simulink library "XXCopter_Control"  (R2015a)
settings: Solver=ode45  SolverMode=SingleTasking  StartTime=0.0  StopTime=10.0  RelTol=1e-3
undefined symbols (not defined in the file or in its folder): a, C_d0, h, h_FA, h_M, I_prop, I_tube, J_FA, J_T, m_FA, m_M, m_prop, Newton, omega_n, R, Raphson, rho, sigma, T_ctrl, theta_0, theta_1, Throtle_TTO_vec, TO_map_Omega, TO_map_Throtle, v_i0, v_i_adim, Vx_adim, Vz_adim, xi
undefined symbols (not defined in the file): direct_feedforward, l, l_arm, Rotation_sign, T_sim
libraries: vrlib x16, XXCopter_Control x10, aerolibutil x3, qcatlib x1, dspinverses x1
(part 1 of 2)
settings Model: Creator=David  LastModifiedBy=David
settings OptimizationCC: BlockReduction=off  BooleanDataType=off
settings DebuggingCC: SaveWithParameterizedLinksMsg=none  UnderspecifiedInitializationDetection=Classic  MergeDetectMultiDrivingBlocksExec=none  SignalResolutionControl=TryResolveAllWithWarning  StrictBusMsg=Warning
settings HardwareCC: TargetUnknown=on

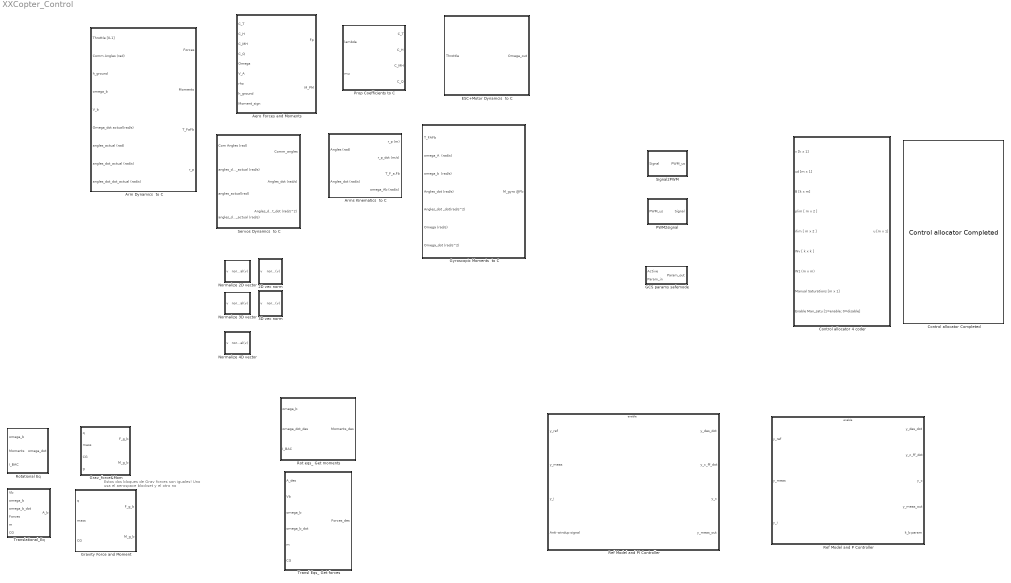
== system XXCopter_Control ==
  note: Estos dos bloques de Grav forces son iguales!
      | Uno usa el aerospace blockset y el otro no
  2D vec norm : Subsystem  TreatAsAtomicUnit=on
  3D vec norm : Subsystem  TreatAsAtomicUnit=on
  "Aero Forces and Moments " : Subsystem  TreatAsAtomicUnit=on
  Arm Dynamics  to C : Subsystem  TreatAsAtomicUnit=on  mask(Arm dynamics, kinematics, forces and moments){Rot_sign=Rotation_sign(1), arm_hub_pos=l*[1;0;0], Arm_axis=[l_arm;0;0], arm_num=1, eta_dir=[1;0;0], gamma_dir=[0;1;0], J_T=J_T, J_FA=J_FA, h=h, switch_val=direct_feedforward, omega_n=35, xi=1.45, eta_inf_lim=deg2rad(-180), eta_sup_lim=deg2rad(180), gamma_inf_lim=deg2rad(-90), gamma_sup_lim=deg2rad(30)}
      mask prompts: Rot_sign "Rotation Sign"; arm_hub_pos "Arm Hub position"; Arm_axis "Arm Hub from servo"; arm_num "Arm number"; eta_dir "eta direcction"; gamma_dir "gamma direction"; J_T "Inertia Motor+prop"; J_FA "Inertia Forearm"; h "h propeller hub"; switch_val "Generation method"; omega_n "Servo natural frequency"; xi "Servo damping"; eta_inf_lim "Pan Servo inf lim (rad)"; eta_sup_lim "Pan Servo sup lim (rad)"; gamma_inf_lim "Tilt Servo inf lim (rad)"; gamma_sup_lim "Tilt servo sup lim  (rad)"
      mask help:
      | This block only accepts arms oriented in x-axis or y-axis: eta and gamma directions can only be [1,0,0] or [0,1,0]
      | Note rotations order is [eta (pan) ,gamma (tilt),0]
      |
      | If Arm number 1 (Forward one)
      | eta_dir=[1,0,0]
      | gamma_dir=[0,1,0]
      |
      | If Arm number 2 or 3 (rear ones)
      | eta_dir=[0,1,0]
      | gamma_dir=[1,0,0]
      mask TypeOptions Rot_sign: Aerodynamics Propeller/Rot_sign | Gyroscopic Moments  to C/Rot_sign
      mask TypeOptions arm_hub_pos: Arms Kinematics  to C/Arm_hub_position
      mask TypeOptions Arm_axis: Gyroscopic Moments  to C/Arm_axis
      mask TypeOptions arm_num: Arms Kinematics  to C/Arm_number
      mask TypeOptions eta_dir: Arms Kinematics  to C/eta_dir | Gyroscopic Moments  to C/eta_dir
      mask TypeOptions gamma_dir: Arms Kinematics  to C/gamma_dir | Gyroscopic Moments  to C/gamma_dir
      mask TypeOptions J_T: Gyroscopic Moments  to C/J_T
      mask TypeOptions J_FA: Gyroscopic Moments  to C/J_FA
      mask TypeOptions h: Arms Kinematics  to C/h_prop
      mask TypeOptions switch_val: Servos Dynamics  to C/switch_val
      mask TypeOptions omega_n: Servos Dynamics  to C/omega_n
      mask TypeOptions xi: Servos Dynamics  to C/xi
      mask TypeOptions eta_inf_lim: Servos Dynamics  to C/eta_inf_lim
      mask TypeOptions eta_sup_lim: Servos Dynamics  to C/eta_sup_lim
      mask TypeOptions gamma_inf_lim: Servos Dynamics  to C/gamma_inf_lim
      mask TypeOptions gamma_sup_lim: Servos Dynamics  to C/gamma_sup_lim
      mask Display:
      | % fprintf(' Arm number %i \n dynamics',arm_num)
      | 
      | 
      | disp(['{\bf \fontsize{16}',sprintf('Arm number\n\n'),num2str(arm_num),sprintf('\n\n Dynamics '),'}'], 'texmode','on');
  Arms Kinematics  to C : Subsystem  TreatAsAtomicUnit=on  mask{Arm_number=1, Arm_hub_position=l*[1;0;0], eta_dir=[1;0;0], gamma_dir=[0;1;0], h_prop=h}
      mask prompts: Arm_number "Arm number (1,2 or 3)"; Arm_hub_position "Arm Hub position"; eta_dir "eta direcction"; gamma_dir "gamma diretion"; h_prop "h of propeller hub"
      mask help:
      | If Arm number 1 (Forward one)
      | eta_dir=[1,0,0]
      | gamma_dir=[0,1,0]
      |
      | If Arm number 2 or 3 (rear ones)
      | eta_dir=[0,1,0]
      | gamma_dir=[1,0,0]
      mask TypeOptions Arm_number: Arm_no/Value
      mask TypeOptions Arm_hub_position: Hub_position/Value
      mask TypeOptions eta_dir: eta_dir/Gain
      mask TypeOptions gamma_dir: gamma_dir/Gain
      mask TypeOptions h_prop: h arm/Value
  Control allocator 4 coder : Subsystem  mask(Control allocator WLS){gamma=1e6, imax=100, T=T_sim}
      mask prompts: gamma "Weight of Control Error Cost (gamma)"; imax "Max # of iterations"; T "Sample Time"
      mask help:
      | Author: David Torres
      | Based on work of Ola Härkegård
  "Control allocator Completed " : qcatlib/Control allocator Completed   alg=WLS  CA_type=QP  iter_max=100  gamma=1  k_B=6  m_B=9  T=T_ctrl  tol=1e-5
  ESC+Motor Dynamcis  to C : Subsystem  TreatAsAtomicUnit=on  VariantControl=Variant_completed
  GCS params safemode : Subsystem  TreatAsAtomicUnit=on
  Grav_force&Mom : Subsystem  TreatAsAtomicUnit=on
  Gravity Force and Moment : MATLAB Function  TreatAsAtomicUnit=on
  Gyroscopic Moments  to C : Subsystem  TreatAsAtomicUnit=on  mask{Arm_axis=[l_arm;0;0], Rot_sign=Rotation_sign(1), eta_dir=[1;0;0], gamma_dir=[0;1;0], J_T=J_T, J_FA=J_FA}
      mask prompts: Arm_axis "Arm axis from Servo origin"; Rot_sign "Rotation sign"; eta_dir "eta direction"; gamma_dir "gamma direction"; J_T "Inertia Motor+Prop"; J_FA "Inertia Foreamr"
      mask TypeOptions Arm_axis: Arm_axis/Value
      mask TypeOptions Rot_sign: Rotation_sign/Value | Rotation_sign1/Value
      mask TypeOptions eta_dir: eta_dir/Gain | eta_dir1/Gain
      mask TypeOptions gamma_dir: gamma_dir/Gain | gamma_dir1/Gain
      mask TypeOptions J_T: Propeller and motor inertia/Value | Propeller and motor inertia1/Value
      mask TypeOptions J_FA: Forearm Inertia/Value | Forearm Inertia1/Value
  Normalize 2D vector : Subsystem  TreatAsAtomicUnit=on
  Normalize 3D vector : Subsystem  TreatAsAtomicUnit=on
  Normalize 4D vector : Subsystem  TreatAsAtomicUnit=on
  PWM2signal : Subsystem  TreatAsAtomicUnit=on  mask{c=2100, a=900, d=1, b=0}
      mask prompts: c "PWM sup limit (us)"; a "PWM inf limit (us)"; d "Signal sup limit"; b "Signal inf limit"
      mask TypeOptions c: up_PWM/Value
      mask TypeOptions a: down_PWM/Value
      mask TypeOptions d: up_signal/Value
      mask TypeOptions b: down_signal/Value
  Prop Coefficients to C : MATLAB Function  TreatAsAtomicUnit=on
  Ref Model and P Controller : Subsystem  mask(Reference Model and Controller){tau=0.2, RisingSlewLimit=4, FallingSlewLimit=-4, K_f=1, K_b=1}
      mask prompts: tau "Desired time constant tau"; RisingSlewLimit "Reference max rising rate"; FallingSlewLimit "Reference max falling rate"; K_f "Rate Feedfordward Gain K_f"; K_b "Proportional Gain K_b"
      mask help:
      | Author: David Torres
      |
      | This block allows a design of the desired dynamics as a 1st order system and the controller of it with P and I actions, with feedforward in rate and anti-windup action.
      |
      |     Inputs: Signal reference, Signal measurement and anti-windup dignal.
      |     Outputs: Desired Signal rate
      |
      | The block shows the expected dynamics assuming the output is integrated with a PERFECT INTEGRATOR or an INTEGRATOR WITH DELAY(delta):
      |      NDI, CA and plant act as a perfect integrator or integrator with a delay delta.
      mask TypeOptions tau: Reference Model/tau
      mask TypeOptions RisingSlewLimit: Rate Limiter/RisingSlewLimit
      mask TypeOptions FallingSlewLimit: Rate Limiter/FallingSlewLimit
      mask TypeOptions K_f: K_f/Gain
      mask TypeOptions K_b: K_b params/Value
      mask Display:
      | K_ref=1/tau;
      | TF = tf([K_ref],[1 K_ref]);
      | 
      | [y,t]=step(TF);
      | S = stepinfo(y,t);
      | 
      | pos = get_param(gcb, 'Position');
      | width = pos(3) - pos(1);
      | height = pos(4) - pos(2);
      | t = t.*width/max(t);
      | y=y.*height/max(y);
      | plot(t,y);
      | S2 = stepinfo(y,t);
      | 
      | if S.Overshoot==0 % 1st order response
      |     text(S2.RiseTime ,height*0.85,['Rise time = ',num2str(S.RiseTime),'s' ]);
      |     text(S2.RiseTime ,height*0.75,['Settling Time = ',num2str(S.SettlingTime)]);
      | 
      | elseif S.Overshoot<0.05 % 2nd order response
      |     text(width*0.5 ,height*0.9,['Rise time = ',num2str(S.RiseTime),'s' ]);
      |     text(width*0.5 ,height*0.8,['Pike time = ',num2str(S.PeakTime),'s' ]);
      |     text(width*0.5 ,height*0.7,['Os = ',num2str(S.Peak)]);
      |     text(width*0.5 ,height*0.6,['SettlingTime = ',num2str(S.SettlingTime)]);
      | else % 2nd order response
      |     text(S2.PeakTime ,S2.Peak*0.85,['Peak time = ',num2str(S.PeakTime),'s' ]);
      |     text(S2.PeakTime ,S2.Peak*0.75,['Os = ',num2str(S.Peak)]);
      |     text(S2.PeakTime ,S2.Peak*0.65,['SettlingTime = ',num2str(S.SettlingTime)]);
      | end
      | 
      | 
      | [num,den] = tfdata(TF);
      | dpoly(num{:},den{:}, 's');
  Ref Model and PI Controller : Subsystem  mask(Reference Model and Controller){delta=0, tau=0.5, RisingSlewLimit=4, FallingSlewLimit=-4, K_f=1, K_a=1, Con_way=auto, omega_n=4, xi=0.5, Z1=-30, K_b=2*0.8*3, f_i=0.25*1/0.8^2, f_c=1}
      mask prompts: delta "Delay on assumed integration: delta (0 for ideal integration)"; tau "Desired time constant tau"; RisingSlewLimit "Reference max rising rate"; FallingSlewLimit "Reference max falling rate"; K_f "Rate Feedfordward Gain"; K_a "Anti-windup gain K_a"; Con_way "Expected response: Controller Design process"; omega_n "Desired 2nd order response omega_n"; xi "Desired 2nd order response  xi"; Z1 "Zero of controller"
      mask help:
      | Author: David Torres
      |
      | This block allows a design of the desired dynamics as a 1st order system and the controller of it with P and I actions, with feedforward in rate and anti-windup action.
      |
      |     Inputs: Signal reference, Signal measurement and anti-windup dignal.
      |     Outputs: Desired Signal rate
      |
      | The block shows the expected dynamics assuming the output is integrated with a PERFECT INTEGRATOR or an INTEGRATOR WITH DELAY(delta):
      |      NDI, CA and plant act as a perfect integrator or integrator with a delay delta.
      mask init:
      | val = get_param(gcb,'MaskValues');
      | K_ref=1/tau;	
      | % Controller design
      | switch lower(val{6})
      |     case 'auto'
      |         K_b=2*xi*omega_n;
      |         f_i=1/(4*xi^2);
      |         if f_i<0.25
      |             f_c = 0.5*(1+sqrt(1-4*f_i));
      |         else
      |             f_c = sqrt(f_i);
      |         end
      |     case 'advanced'
      |         K_b=2*xi*omega_n;
      |         f_i=1/(4*xi^2);
      |         f_c =  -omega_n/(2*xi*Z1);  
      |     case 'pro'
      | end
      mask TypeOptions delta: PI Controller/delta
      mask TypeOptions tau: Reference Model/tau
      mask TypeOptions RisingSlewLimit: Rate Limiter/RisingSlewLimit
      mask TypeOptions FallingSlewLimit: Rate Limiter/FallingSlewLimit
      mask TypeOptions K_f: K_f/Gain
      mask TypeOptions K_a: PI Controller/K_a
      mask TypeOptions Con_way: auto | advanced | pro
      mask Callback Con_way:
      | val = get_param(gcb,'MaskValues');
      | switch lower(val{6})
      |  case 'auto'
      |      set_param(gcb,'MaskVisibilities',{'on','on','on','on','on','on','on','on','off','off','off','off'});
      |  case 'advanced'
      |      set_param(gcb,'MaskVisibilities',{'on','on','on','on','on','on','on','on','on','off','off','off'});
      |  case 'pro'
      |      set_param(gcb,'MaskVisibilities',{'on','on','on','on','on','on','off','off','off','on','on','on'});
      |  end
      mask TypeOptions K_b: PI Controller/K_b
      mask TypeOptions f_i: PI Controller/f_i
      mask TypeOptions f_c: PI Controller/f_c
      mask Display:
      | RM = tf([K_ref],[1 K_ref]);
      | 
      | if delta==0
      |     TF_FF = tf([K_f K_b*f_c K_b*f_i*K_b],[1 K_b f_i*K_b^2]);
      | else
      |     s=tf('s');
      |     TF_FF = 1/(s+delta)*(K_f*s^2+K_b*(f_c*s+f_i*K_b))/(s + 1/(s+delta)*(K_b*s+f_i*K_b^2) );
      | end
      | TF = RM*TF_FF;
      | 
      | [y,t]=step(TF);
      | S = stepinfo(y,t);
      | 
      | pos = get_param(gcb, 'Position');
      | width = pos(3) - pos(1);
      | height = pos(4) - pos(2);
      | t = t.*width/max(t);
      | y=y.*height/max(y);
      | plot(t,y);
      | S2 = stepinfo(y,t);
      | 
      | if S.Overshoot==0 % 1st order response
      |     text(S2.RiseTime ,height*0.85,['Rise time = ',num2str(S.RiseTime),'s' ]);
      |     text(S2.RiseTime ,height*0.75,['Settling Time = ',num2str(S.SettlingTime)]);
      | 
      | elseif S.Overshoot<0.05 % 2nd order response
      |     text(width*0.5 ,height*0.9,['Rise time = ',num2str(S.RiseTime),'s' ]);
      |     text(width*0.5 ,height*0.8,['Pike time = ',num2str(S.PeakTime),'s' ]);
      |     text(width*0.5 ,height*0.7,['Os = ',num2str(S.Peak)]);
      |     text(width*0.5 ,height*0.6,['SettlingTime = ',num2str(S.SettlingTime)]);
      | else % 2nd order response
      |     text(S2.PeakTime ,S2.Peak*0.85,['Peak time = ',num2str(S.PeakTime),'s' ]);
      |     text(S2.PeakTime ,S2.Peak*0.75,['Os = ',num2str(S.Peak)]);
      |     text(S2.PeakTime ,S2.Peak*0.65,['SettlingTime = ',num2str(S.SettlingTime)]);
      | end
      | 
      | text(0.1*width,0.1*height,['EXPECTED CLOSED-LOOP RESPONSE: INTEGRATION DELAY OF ',num2str(delta),'s ']);
      | 
      | [num,den] = tfdata(TF);
      | dpoly(num{:},den{:}, 's');
  Rot eqs_ Get moments : Subsystem  TreatAsAtomicUnit=on
  Rotational Eq : Subsystem  TreatAsAtomicUnit=on
  Servos Dynamics  to C : Subsystem  TreatAsAtomicUnit=on  mask{switch_val=direct_feedforward, omega_n=omega_n, xi=xi, eta_inf_lim=-0.5, eta_sup_lim=0.5, gamma_inf_lim=-0.5, gamma_sup_lim=0.5}
      mask prompts: switch_val "Generation method"; omega_n "Servo natural freq (rad/s) omega_n"; xi "Servo damping xi"; eta_inf_lim "Pan Servo inf lim"; eta_sup_lim "Pan servo sup lim"; gamma_inf_lim "Tilt servo inf lim"; gamma_sup_lim "Tilt servo sup lim"
      mask init:
      | val = get_param(gcb,'MaskValues');
      | switch lower(val{1})
      |  case 'properties_based'
      |      switch_val=0;
      |  case 'direct_feedforward'
      |      switch_val=1;
      | end
      mask TypeOptions switch_val: properties_based | direct_feedforward
      mask Callback switch_val:
      | val = get_param(gcb,'MaskValues');
      | switch lower(val{1})
      |  case 'properties_based'
      |      switch_val=0;
      |  case 'direct_feedforward'
      |      switch_val=1;
      | end
      mask TypeOptions omega_n: omega_n/Value
      mask TypeOptions xi: xi/Value
      mask TypeOptions eta_inf_lim: pan_lim/LowerLimit
      mask TypeOptions eta_sup_lim: pan_lim/UpperLimit
      mask TypeOptions gamma_inf_lim: tilt_lim/LowerLimit
      mask TypeOptions gamma_sup_lim: tilt_lim/UpperLimit
  Signal2PWM : Subsystem  TreatAsAtomicUnit=on  mask{b=1, d=0, a=2100, c=900}
      mask prompts: b "Signal sup limit"; d "Signal inf limit"; a "PWM sup limit (us)"; c "PWM inf limit (us)"
      mask TypeOptions b: up_signal/Value
      mask TypeOptions d: down_signal/Value
      mask TypeOptions a: up_PWM/Value
      mask TypeOptions c: down_PWM/Value
  Transl Eqs_ Get forces : Subsystem  TreatAsAtomicUnit=on
  Translational_Eq : Subsystem  TreatAsAtomicUnit=on

== system XXCopter_Control/2D vec norm ==
  v : Inport
  norm^2rm : Subsystem  TreatAsAtomicUnit=on
  sqrt : Sqrt  AlgorithmType=Newton-Raphson  SaturateOnIntegerOverflow=on
  norm(v) : Outport
  wires:
  sqrt/1 -> norm(v)/1
  norm^2rm/1(norm(v)) -> sqrt/1
  v/1 -> norm^2rm/1(v)

== system XXCopter_Control/3D vec norm ==
  v : Inport
  norm^2rm : Subsystem  TreatAsAtomicUnit=on
  sqrt : Sqrt  AlgorithmType=Newton-Raphson  SaturateOnIntegerOverflow=on
  norm(v) : Outport
  wires:
  v/1 -> norm^2rm/1(v)
  norm^2rm/1(norm(v)) -> sqrt/1
  sqrt/1 -> norm(v)/1

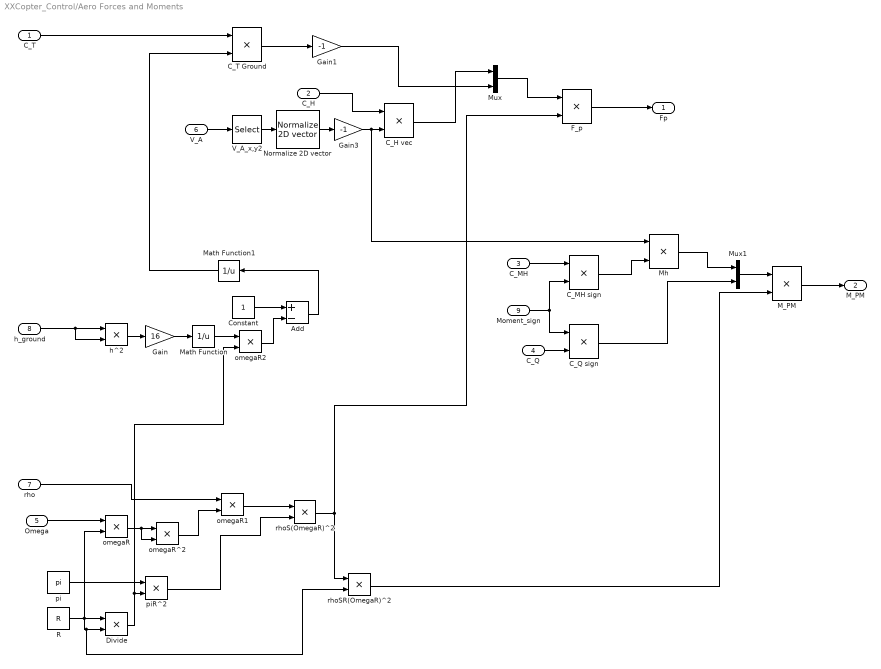
== system XXCopter_Control/Aero Forces and Moments  ==
  C_T : Inport
  C_H : Inport  Port=2
  C_MH : Inport  Port=3
  C_Q : Inport  Port=4
  Omega : Inport  Port=5
  V_A : Inport  Port=6
  rho : Inport  Port=7
  h_ground : Inport  Port=8
  Moment_sign : Inport  Port=9
  Add : Sum  Inputs=+-
  C_H vec : Product  Inputs=**
  C_MH sign : Product  Inputs=**
  C_Q sign : Product  Inputs=**
  C_T Ground : Product  Inputs=**
  Constant : Constant
  Divide : Product  Inputs=**
  F_p : Product  Inputs=**
  Gain : Gain  Gain=16
  Gain1 : Gain  Gain=-1
  Gain3 : Gain  Gain=-1
  M_PM : Product  Inputs=**
  Math Function : Math  Operator=reciprocal  SaturateOnIntegerOverflow=on
  Math Function1 : Math  Operator=reciprocal  SaturateOnIntegerOverflow=on
  Mh : Product  Inputs=**
  Mux : Mux  Inputs=[2,1]
  Mux1 : Mux  Inputs=[2,1]
  Normalize 2D vector : XXCopter_Control/Normalize 2D vector
  R : Constant  Value=R
  V_A_x,y2 : Selector  IndexMode=Zero-based  InputPortWidth=3  Indices=[0,1]
  h^2 : Product  Inputs=**
  omegaR : Product  Inputs=**
  omegaR1 : Product  Inputs=**
  omegaR2 : Product  Inputs=**
  omegaR^2 : Product  Inputs=**
  pi : Constant  Value=pi
  piR^2 : Product  Inputs=**
  rhoS(OmegaR)^2 : Product  Inputs=**
  rhoSR(OmegaR)^2 : Product  Inputs=**
  Fp : Outport
  "M_PM " : Outport  Port=2
  wires:
  R/1 -> rhoSR(OmegaR)^2/2, Divide/2, omegaR/2, Divide/1
  pi/1 -> piR^2/1
  Divide/1 -> omegaR2/2, piR^2/2
  Omega/1 -> omegaR/1
  rho/1 -> omegaR1/1
  omegaR/1 -> omegaR^2/2, omegaR^2/1
  omegaR^2/1 -> omegaR1/2
  piR^2/1 -> rhoS(OmegaR)^2/2
  omegaR1/1 -> rhoS(OmegaR)^2/1
  C_T/1 -> C_T Ground/1
  h_ground/1 -> h^2/2, h^2/1
  h^2/1 -> Gain/1
  Gain/1 -> Math Function/1
  Math Function/1 -> omegaR2/1
  Constant/1 -> Add/1
  omegaR2/1 -> Add/2
  Add/1 -> Math Function1/1
  Math Function1/1 -> C_T Ground/2
  C_T Ground/1 -> Gain1/1
  V_A_x,y2/1 -> Normalize 2D vector/1
  V_A/1 -> V_A_x,y2/1
  Normalize 2D vector/1 -> Gain3/1
  Gain3/1 -> Mh/1, C_H vec/2
  C_H/1 -> C_H vec/1
  C_H vec/1 -> Mux/1
  Gain1/1 -> Mux/2
  Mux/1 -> F_p/1
  rhoS(OmegaR)^2/1 -> rhoSR(OmegaR)^2/1, F_p/2
  C_MH/1 -> C_MH sign/1
  Moment_sign/1 -> C_MH sign/2, C_Q sign/1
  C_MH sign/1 -> Mh/2
  Mh/1 -> Mux1/1
  F_p/1 -> Fp/1
  Mux1/1 -> M_PM/1
  C_Q/1 -> C_Q sign/2
  C_Q sign/1 -> Mux1/2
  rhoSR(OmegaR)^2/1 -> M_PM/2
  M_PM/1 -> "M_PM "/1

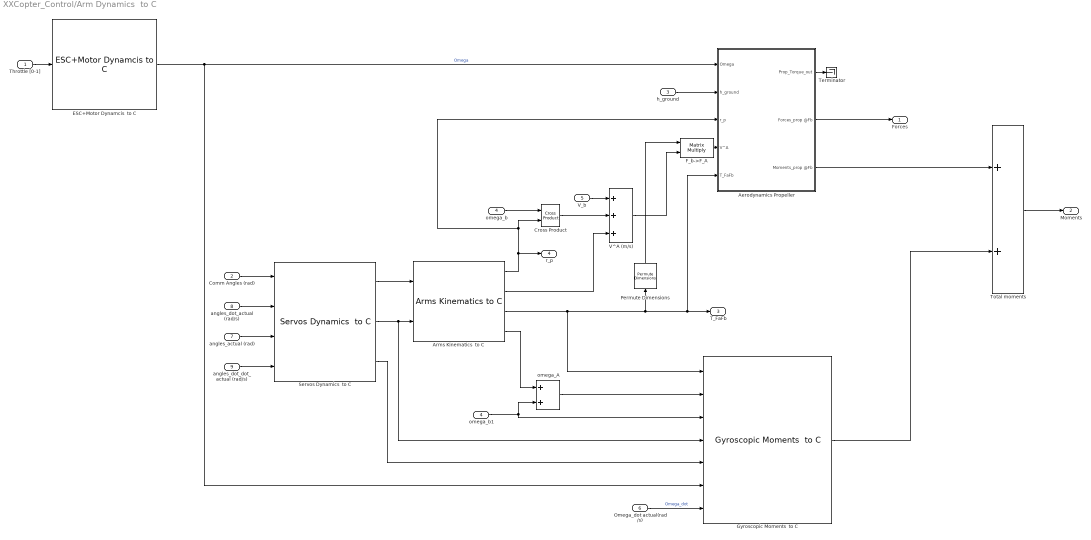
== system XXCopter_Control/Arm Dynamics  to C ==
  Throttle [0-1] : Inport
  Comm Angles (rad) : Inport  Port=2
  h_ground : Inport  Port=3
  omega_b : Inport  Port=4
  V_b : Inport  Port=5
  Omega_dot actual(rad/s) : Inport  Port=6
  angles_actual (rad) : Inport  Port=7
  angles_dot_actual (rad/s) : Inport  Port=8
  angles_dot_dot_actual (rad/s) : Inport  Port=9
  Aerodynamics Propeller : Subsystem  TreatAsAtomicUnit=on  mask{Rot_sign=Rot_sign}
      mask prompts: Rot_sign "Rotation Sign"
      settings: MinAlgLoopOccurrences=on
      mask TypeOptions Rot_sign: Rotation_sign/Value
  Arms Kinematics  to C : XXCopter_Control/Arms Kinematics  to C  Arm_number=arm_num  Arm_hub_position=arm_hub_pos  eta_dir=eta_dir  gamma_dir=gamma_dir  h_prop=h
  Cross Product : vrlib/Utilities/Cross Product
  ESC+Motor Dynamcis  to C : XXCopter_Control/ESC+Motor Dynamcis  to C  VariantControl=Variant_completed
  F_b->F_A : Product  Multiplication=Matrix(*)
  Gyroscopic Moments  to C : XXCopter_Control/Gyroscopic Moments  to C  Arm_axis=Arm_axis  Rot_sign=Rot_sign  eta_dir=eta_dir  gamma_dir=gamma_dir  J_T=J_T  J_FA=J_FA
  Permute Dimensions : PermuteDimensions
  Servos Dynamics  to C : XXCopter_Control/Servos Dynamics  to C  switch_val=direct_feedforward  omega_n=omega_n  xi=xi  eta_inf_lim=eta_inf_lim  eta_sup_lim=eta_sup_lim  gamma_inf_lim=gamma_inf_lim  gamma_sup_lim=gamma_sup_lim
  Terminator : Terminator
  Total moments : Sum
  V^A (m/s) : Sum  Inputs=+++
  omega_A : Sum
  omega_b1 : InportShadow  Port=4
  Forces : Outport
  Moments : Outport  Port=2
  T_FaFb : Outport  Port=3
  r_p : Outport  Port=4
  wires:
  Throttle [0-1]/1 -> ESC+Motor Dynamcis  to C/1
  Omega_dot actual(rad/s)/1 -> Gyroscopic Moments  to C/7  "Omega_dot"
  ESC+Motor Dynamcis  to C/1 -> Gyroscopic Moments  to C/6, Aerodynamics Propeller/1(Omega)  "Omega"
  h_ground/1 -> Aerodynamics Propeller/2(h_ground)
  Comm Angles (rad)/1 -> Servos Dynamics  to C/1
  omega_b/1 -> Cross Product/1
  Cross Product/1 -> V^A (m/s)/2
  V_b/1 -> V^A (m/s)/1
  Arms Kinematics  to C/2 -> V^A (m/s)/3
  Arms Kinematics  to C/1 -> Aerodynamics Propeller/3(r_p), Cross Product/2, r_p/1
  Aerodynamics Propeller/2(Forces_prop @Fb) -> Forces/1
  Servos Dynamics  to C/2 -> Gyroscopic Moments  to C/4, Arms Kinematics  to C/2
  Arms Kinematics  to C/4 -> omega_A/1
  omega_b1/1 -> Gyroscopic Moments  to C/3, omega_A/2
  omega_A/1 -> Gyroscopic Moments  to C/2
  angles_dot_actual (rad/s)/1 -> Servos Dynamics  to C/2
  Aerodynamics Propeller/3(Moments_prop @Fb) -> Total moments/1
  Gyroscopic Moments  to C/1 -> Total moments/2
  Total moments/1 -> Moments/1
  angles_actual (rad)/1 -> Servos Dynamics  to C/3
  Aerodynamics Propeller/1(Prop_Torque_out) -> Terminator/1
  Servos Dynamics  to C/1 -> Arms Kinematics  to C/1
  Servos Dynamics  to C/3 -> Gyroscopic Moments  to C/5
  angles_dot_dot_actual (rad/s)/1 -> Servos Dynamics  to C/4
  Arms Kinematics  to C/3 -> Gyroscopic Moments  to C/1, Permute Dimensions/1, Aerodynamics Propeller/5(T_FaFb), T_FaFb/1
  V^A (m/s)/1 -> F_b->F_A/2
  Permute Dimensions/1 -> F_b->F_A/1
  F_b->F_A/1 -> Aerodynamics Propeller/4(V^A)

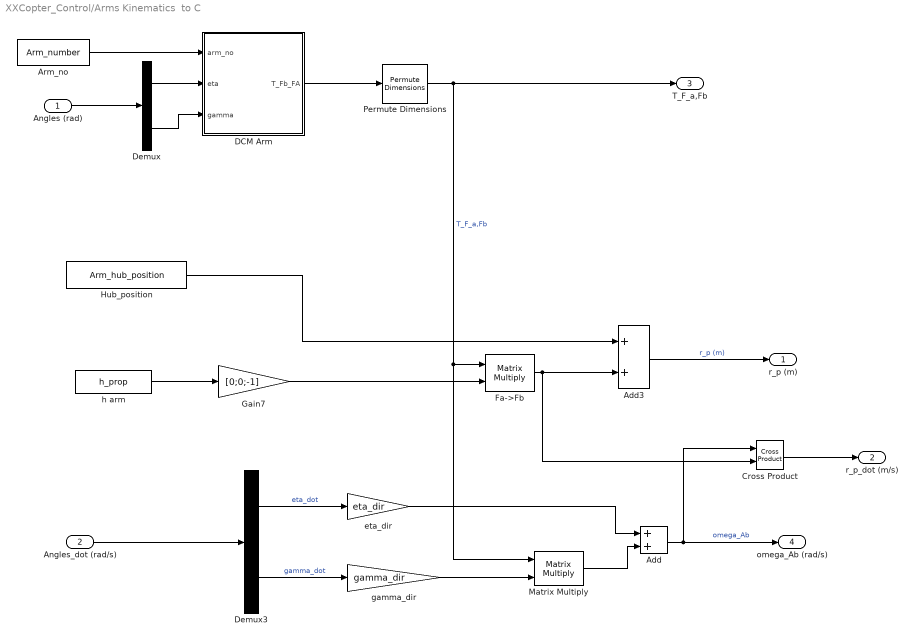
== system XXCopter_Control/Arms Kinematics  to C ==
  Angles (rad) : Inport
  Angles_dot (rad/s) : Inport  Port=2
  Add : Sum
  Add3 : Sum
  Arm_no : Constant  Value=Arm_number
  Cross Product : vrlib/Utilities/Cross Product
  DCM Arm : MATLAB Function  TreatAsAtomicUnit=on
  Demux : Demux  Outputs=2
  Demux3 : Demux  Outputs=2
  Fa->Fb : Product  Multiplication=Matrix(*)
  Gain7 : Gain  Gain=[0;0;-1]
  Hub_position : Constant  Value=Arm_hub_position
  Matrix Multiply : Product  Multiplication=Matrix(*)
  Permute Dimensions : PermuteDimensions
  eta_dir : Gain  Gain=eta_dir
  gamma_dir : Gain  Gain=gamma_dir
  h arm : Constant  Value=h_prop
  r_p (m) : Outport
  r_p_dot (m/s) : Outport  Port=2
  T_F_a,Fb : Outport  Port=3
  omega_Ab (rad/s) : Outport  Port=4
  wires:
  DCM Arm/1(T_Fb_FA) -> Permute Dimensions/1
  Permute Dimensions/1 -> T_F_a,Fb/1, Matrix Multiply/1, Fa->Fb/1  "T_F_a,Fb"
  Angles (rad)/1 -> Demux/1
  Demux/1 -> DCM Arm/2(eta)
  Demux/2 -> DCM Arm/3(gamma)
  Angles_dot (rad/s)/1 -> Demux3/1
  Demux3/2 -> gamma_dir/1  "gamma_dot"
  Demux3/1 -> eta_dir/1  "eta_dot"
  gamma_dir/1 -> Matrix Multiply/2
  Matrix Multiply/1 -> Add/2
  eta_dir/1 -> Add/1
  Add/1 -> Cross Product/1, omega_Ab (rad/s)/1  "omega_Ab"
  Add3/1 -> r_p (m)/1  "r_p (m)"
  h arm/1 -> Gain7/1
  Gain7/1 -> Fa->Fb/2
  Hub_position/1 -> Add3/1
  Fa->Fb/1 -> Cross Product/2, Add3/2
  Cross Product/1 -> r_p_dot (m/s)/1
  Arm_no/1 -> DCM Arm/1(arm_no)

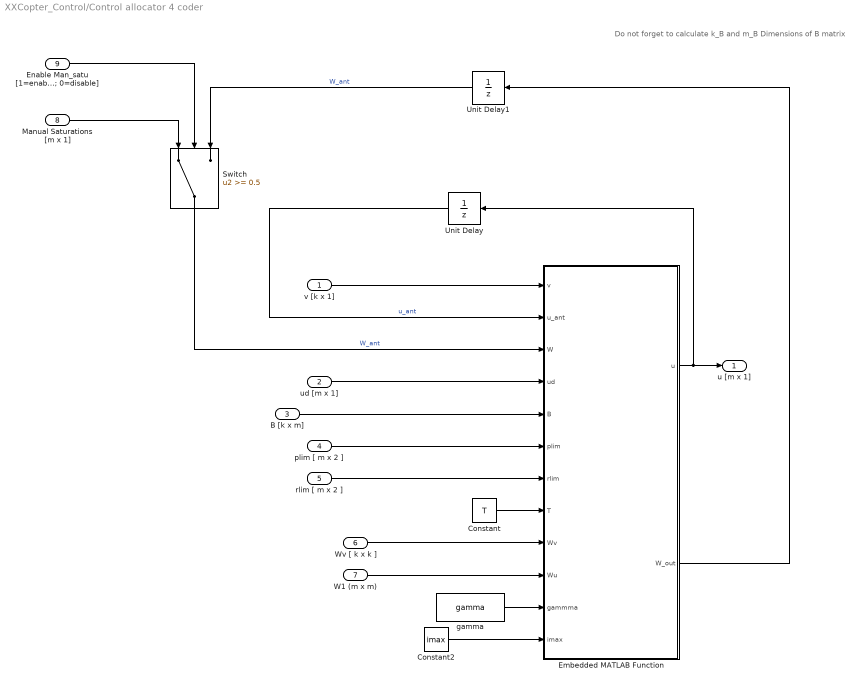
== system XXCopter_Control/Control allocator 4 coder ==
  note: Do not forget to calculate k_B and m_B Dimensions of B matrix
  v [k x 1] : Inport
  ud [m x 1] : Inport  Port=2
  B [k x m] : Inport  Port=3
  plim [ m x 2 ] : Inport  Port=4
  rlim [ m x 2 ] : Inport  Port=5
  Wv [ k x k ] : Inport  Port=6
  W1 (m x m) : Inport  Port=7
  Manual Saturations [m x 1] : Inport  Port=8
  Enable Man_satu [1=enable; 0=disable] : Inport  Port=9
  Constant : Constant  Value=T
  Constant2 : Constant  Value=imax
  Embedded MATLAB Function : MATLAB Function  TreatAsAtomicUnit=on
  Switch : Switch  Threshold=0.5  SampleTime=T
  Unit Delay : UnitDelay  InitialCondition=zeros(9,1)  SampleTime=T
  Unit Delay1 : UnitDelay  InitialCondition=zeros(9,1)  SampleTime=T
  gamma : Constant  Value=gamma
  u [m x 1] : Outport
  wires:
  Enable Man_satu [1=enable; 0=disable]/1 -> Switch/2
  Manual Saturations [m x 1]/1 -> Switch/1
  Unit Delay1/1 -> Switch/3  "W_ant"
  Embedded MATLAB Function/1(u) -> Unit Delay/1, u [m x 1]/1
  Switch/1 -> Embedded MATLAB Function/3(W)  "W_ant"
  Embedded MATLAB Function/2(W_out) -> Unit Delay1/1
  ud [m x 1]/1 -> Embedded MATLAB Function/4(ud)
  W1 (m x m)/1 -> Embedded MATLAB Function/10(Wu)
  Wv [ k x k ]/1 -> Embedded MATLAB Function/9(Wv)
  rlim [ m x 2 ]/1 -> Embedded MATLAB Function/7(rlim)
  plim [ m x 2 ]/1 -> Embedded MATLAB Function/6(plim)
  B [k x m]/1 -> Embedded MATLAB Function/5(B)
  Unit Delay/1 -> Embedded MATLAB Function/2(u_ant)  "u_ant"
  v [k x 1]/1 -> Embedded MATLAB Function/1(v)
  Constant/1 -> Embedded MATLAB Function/8(T)
  gamma/1 -> Embedded MATLAB Function/11(gammma)
  Constant2/1 -> Embedded MATLAB Function/12(imax)

== system XXCopter_Control/ESC+Motor Dynamcis  to C ==
  Throttle : Inport
  2-D Torque-Throttle-Omega Map : Lookup_n-D  NumberOfTableDimensions=1  BreakpointsForDimension1=TO_map_Throtle  BreakpointsForDimension2=Throtle_TTO_vec  Table=TO_map_Omega  TableDataTypeStr=single  IntermediateResultsDataTypeStr=single  ExtrapMethod=Clip  DiagnosticForOutOfRangeInput=Warning  RemoveProtectionInput=on  OutDataTypeStr=single  RndMeth=Zero  FractionDataTypeStr=single  InputSameDT=on
  Bias : Bias  Bias=eps
  Omega_out : Outport
  wires:
  2-D Torque-Throttle-Omega Map/1 -> Bias/1
  Bias/1 -> Omega_out/1
  Throttle/1 -> 2-D Torque-Throttle-Omega Map/1

== system XXCopter_Control/GCS params safemode ==
  Active : Inport
  Param_in : Inport  Port=2
  Data Type Conversion : DataTypeConversion  OutDataTypeStr=boolean
  Delay : Delay  DelayLength=5  InitialCondition=0
  Logical Operator : Logic  IconShape=distinctive  AllPortsSameDT=off  OutDataTypeStr=boolean
  Relational Operator : RelationalOperator  Operator=~=  OutDataTypeStr=boolean
  Sample&Hold : Subsystem  TreatAsAtomicUnit=on
  Unit Delay : UnitDelay  SampleTime=-1
  Param_out : Outport
  wires:
  Param_in/1 -> Sample&Hold/1(In1), Relational Operator/1, Unit Delay/1
  Unit Delay/1 -> Relational Operator/2
  Relational Operator/1 -> Logical Operator/2
  Active/1 -> Delay/1
  Data Type Conversion/1 -> Logical Operator/1
  Logical Operator/1 -> Sample&Hold/Trigger
  Sample&Hold/1(Out1) -> Param_out/1
  Delay/1 -> Data Type Conversion/1

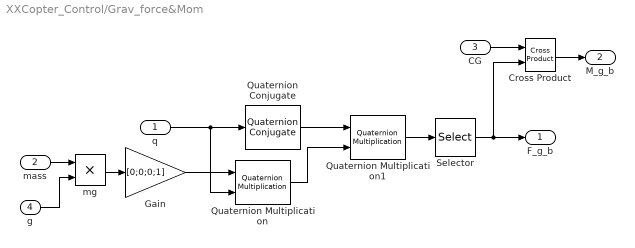
== system XXCopter_Control/Grav_force&Mom ==
  q : Inport
  mass : Inport  Port=2
  CG : Inport  Port=3
  g : Inport  Port=4
  Cross Product : vrlib/Utilities/Cross Product
  Gain : Gain  Gain=[0;0;0;1]
  Quaternion Conjugate : aerolibutil/Quaternion Conjugate
  Quaternion Multiplication : aerolibutil/Quaternion Multiplication
  Quaternion Multiplication1 : aerolibutil/Quaternion Multiplication
  Selector : Selector  IndexMode=Zero-based  InputPortWidth=4  Indices=[1:3]
  mg : Product  RndMeth=Zero
  F_g_b : Outport
  M_g_b : Outport  Port=2
  wires:
  mass/1 -> mg/1
  g/1 -> mg/2
  mg/1 -> Gain/1
  Gain/1 -> Quaternion Multiplication/1
  q/1 -> Quaternion Conjugate/1, Quaternion Multiplication/2
  Quaternion Conjugate/1 -> Quaternion Multiplication1/1
  Quaternion Multiplication/1 -> Quaternion Multiplication1/2
  Quaternion Multiplication1/1 -> Selector/1
  Selector/1 -> Cross Product/2, F_g_b/1
  CG/1 -> Cross Product/1
  Cross Product/1 -> M_g_b/1

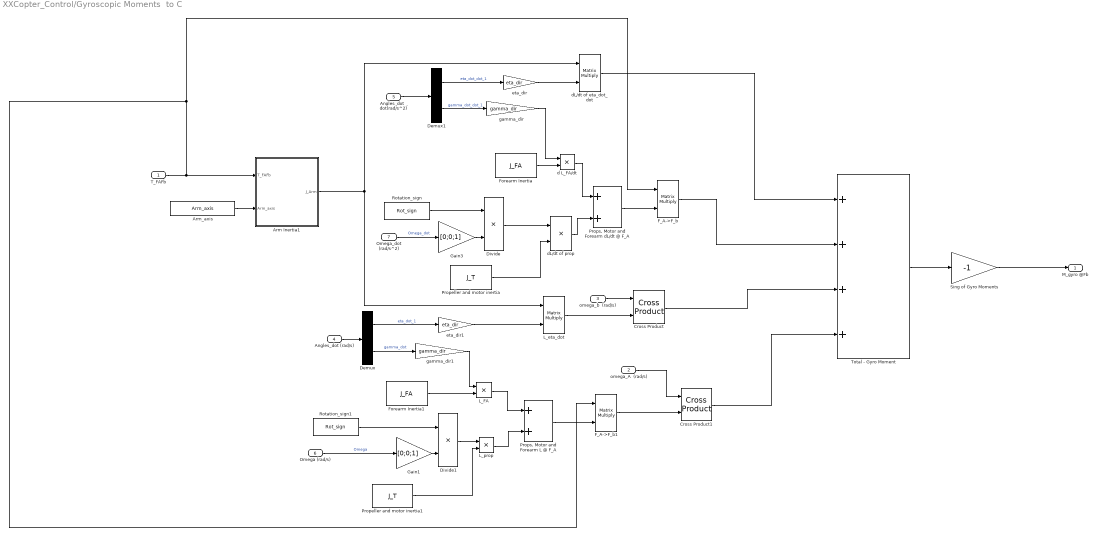
== system XXCopter_Control/Gyroscopic Moments  to C ==
  T_FAFb : Inport
  omega_A  (rad/s) : Inport  Port=2
  omega_b  (rad/s) : Inport  Port=3
  Angles_dot (rad/s) : Inport  Port=4
  Angles_dot _dot(rad/s^2) : Inport  Port=5
  Omega (rad/s) : Inport  Port=6
  Omega_dot (rad/s^2) : Inport  Port=7
  Arm Inertia1 : MATLAB Function  TreatAsAtomicUnit=on
  Arm_axis : Constant  Value=Arm_axis
  Cross Product : vrlib/Utilities/Cross Product
  Cross Product1 : vrlib/Utilities/Cross Product
  Demux : Demux  Outputs=2
  Demux1 : Demux  Outputs=2
  Divide : Product  Inputs=**
  Divide1 : Product  Inputs=**
  F_A->F_b : Product  Multiplication=Matrix(*)
  F_A->F_b1 : Product  Multiplication=Matrix(*)
  Forearm Inertia : Constant  Value=J_FA
  Forearm Inertia1 : Constant  Value=J_FA
  Gain1 : Gain  Gain=[0;0;1]
  Gain3 : Gain  Gain=[0;0;1]
  L_FA : Product  Inputs=**
  L_eta_dot : Product  Multiplication=Matrix(*)
  L_prop : Product  Inputs=**
  Propeller and motor inertia : Constant  Value=J_T
  Propeller and motor inertia1 : Constant  Value=J_T
  "Props, Motor and Forearm L @ F_A" : Sum
  "Props, Motor and Forearm dL/dt @ F_A" : Sum
  Rotation_sign : Constant  Value=Rot_sign
  Rotation_sign1 : Constant  Value=Rot_sign
  Sing of Gyro Moments : Gain  Gain=-1
  Total - Gyro Moment : Sum  Inputs=++++
  d L_FA/dt : Product  Inputs=**
  dL/dt of eta_dot_dot : Product  Multiplication=Matrix(*)
  dL/dt of prop : Product  Inputs=**
  eta_dir : Gain  Gain=eta_dir
  eta_dir1 : Gain  Gain=eta_dir
  gamma_dir : Gain  Gain=gamma_dir
  gamma_dir1 : Gain  Gain=gamma_dir
  M_gyro @Fb : Outport
  wires:
  Angles_dot (rad/s)/1 -> Demux/1
  Angles_dot _dot(rad/s^2)/1 -> Demux1/1
  Demux1/1 -> eta_dir/1  "eta_dot_dot_1"
  Arm Inertia1/1(J_Arm) -> L_eta_dot/1, dL/dt of eta_dot_dot/1
  eta_dir/1 -> dL/dt of eta_dot_dot/2
  eta_dir1/1 -> L_eta_dot/2
  Demux/1 -> eta_dir1/1  "eta_dot_1"
  L_eta_dot/1 -> Cross Product/2
  omega_b  (rad/s)/1 -> Cross Product/1
  Demux1/2 -> gamma_dir/1  "gamma_dot_dot_1"
  gamma_dir/1 -> d L_FA/dt/1
  Forearm Inertia/1 -> d L_FA/dt/2
  Omega_dot (rad/s^2)/1 -> Gain3/1  "Omega_dot"
  Divide/1 -> dL/dt of prop/1
  Propeller and motor inertia/1 -> dL/dt of prop/2
  d L_FA/dt/1 -> "Props, Motor and Forearm dL/dt @ F_A"/1
  dL/dt of prop/1 -> "Props, Motor and Forearm dL/dt @ F_A"/2
  Demux/2 -> gamma_dir1/1  "gamma_dot"
  gamma_dir1/1 -> L_FA/1
  Forearm Inertia1/1 -> L_FA/2
  Divide1/1 -> L_prop/1
  Propeller and motor inertia1/1 -> L_prop/2
  L_FA/1 -> "Props, Motor and Forearm L @ F_A"/1
  L_prop/1 -> "Props, Motor and Forearm L @ F_A"/2
  Omega (rad/s)/1 -> Gain1/1  "Omega"
  "Props, Motor and Forearm dL/dt @ F_A"/1 -> F_A->F_b/2
  F_A->F_b/1 -> Total - Gyro Moment/2
  dL/dt of eta_dot_dot/1 -> Total - Gyro Moment/1
  Cross Product/1 -> Total - Gyro Moment/3
  "Props, Motor and Forearm L @ F_A"/1 -> F_A->F_b1/2
  T_FAFb/1 -> Arm Inertia1/1(T_FAFb), F_A->F_b/1, F_A->F_b1/1
  F_A->F_b1/1 -> Cross Product1/2
  omega_A  (rad/s)/1 -> Cross Product1/1
  Cross Product1/1 -> Total - Gyro Moment/4
  Total - Gyro Moment/1 -> Sing of Gyro Moments/1
  Sing of Gyro Moments/1 -> M_gyro @Fb/1
  Arm_axis/1 -> Arm Inertia1/2(Arm_axis)
  Rotation_sign/1 -> Divide/1
  Gain3/1 -> Divide/2
  Rotation_sign1/1 -> Divide1/1
  Gain1/1 -> Divide1/2

== system XXCopter_Control/Normalize 2D vector ==
  v : Inport
  2D vec norm : XXCopter_Control/2D vec norm
  Bias : Bias  Bias=eps
  Demux : Demux  Outputs=2
  Math Function : Math  Operator=reciprocal  SaturateOnIntegerOverflow=on
  Mux : Mux  Inputs=2
  Product2 : Product  Inputs=**
  Product3 : Product  Inputs=**
  normal(v) : Outport
  wires:
  Math Function/1 -> Product2/2, Product3/2
  Demux/2 -> Product3/1
  Demux/1 -> Product2/1
  Mux/1 -> normal(v)/1
  v/1 -> 2D vec norm/1, Demux/1
  Bias/1 -> Math Function/1
  Product2/1 -> Mux/1
  Product3/1 -> Mux/2
  2D vec norm/1 -> Bias/1

== system XXCopter_Control/Normalize 3D vector ==
  v : Inport
  3D vec norm : XXCopter_Control/3D vec norm
  Bias : Bias  Bias=eps
  Demux : Demux  Outputs=3
  Math Function : Math  Operator=reciprocal  SaturateOnIntegerOverflow=on
  Mux : Mux  Inputs=3
  Product1 : Product  Inputs=**
  Product2 : Product  Inputs=**
  Product3 : Product  Inputs=**
  normal(v) : Outport
  wires:
  Demux/2 -> Product3/1
  Demux/1 -> Product2/1
  Mux/1 -> normal(v)/1
  v/1 -> 3D vec norm/1, Demux/1
  3D vec norm/1 -> Bias/1
  Product2/1 -> Mux/1
  Product3/1 -> Mux/2
  Demux/3 -> Product1/1
  Math Function/1 -> Product2/2, Product3/2, Product1/2
  Product1/1 -> Mux/3
  Bias/1 -> Math Function/1

== system XXCopter_Control/Normalize 4D vector ==
  v : Inport
  4D vec norm : Subsystem  TreatAsAtomicUnit=on
  Bias : Bias  Bias=eps
  Demux : Demux
  Math Function : Math  Operator=reciprocal  SaturateOnIntegerOverflow=on
  Mux : Mux
  Product{1..4} (4 alike) : Product  Inputs=**
  normal(v) : Outport
  wires:
  Bias/1 -> Math Function/1
  Product1/1 -> Mux/3
  Math Function/1 -> Product4/2, Product1/2, Product3/2, Product2/2
  Demux/3 -> Product1/1
  Product3/1 -> Mux/2
  Product2/1 -> Mux/1
  4D vec norm/1(norm(v)) -> Bias/1
  v/1 -> 4D vec norm/1(v), Demux/1
  Mux/1 -> normal(v)/1
  Demux/1 -> Product2/1
  Demux/2 -> Product3/1
  Demux/4 -> Product4/1
  Product4/1 -> Mux/4

== system XXCopter_Control/PWM2signal ==
  PWM_us : Inport
  Add : Sum  Inputs=+-
  Add1 : Sum  Inputs=+-
  Add2 : Sum  Inputs=+-
  Add3 : Sum
  Divide : Product  Inputs=*/
  Divide1 : Product  Inputs=**
  down_PWM : Constant  Value=a
  down_signal : Constant  Value=b
  up_PWM : Constant  Value=c
  up_signal : Constant  Value=d
  Signal : Outport
  wires:
  Add3/1 -> Signal/1
  Divide1/1 -> Add3/2
  Add2/1 -> Divide1/1
  Divide/1 -> Divide1/2
  down_signal/1 -> Add2/2, Add3/1
  up_signal/1 -> Add2/1
  Add/1 -> Divide/1
  Add1/1 -> Divide/2
  up_PWM/1 -> Add1/1
  down_PWM/1 -> Add1/2, Add/2
  PWM_us/1 -> Add/1

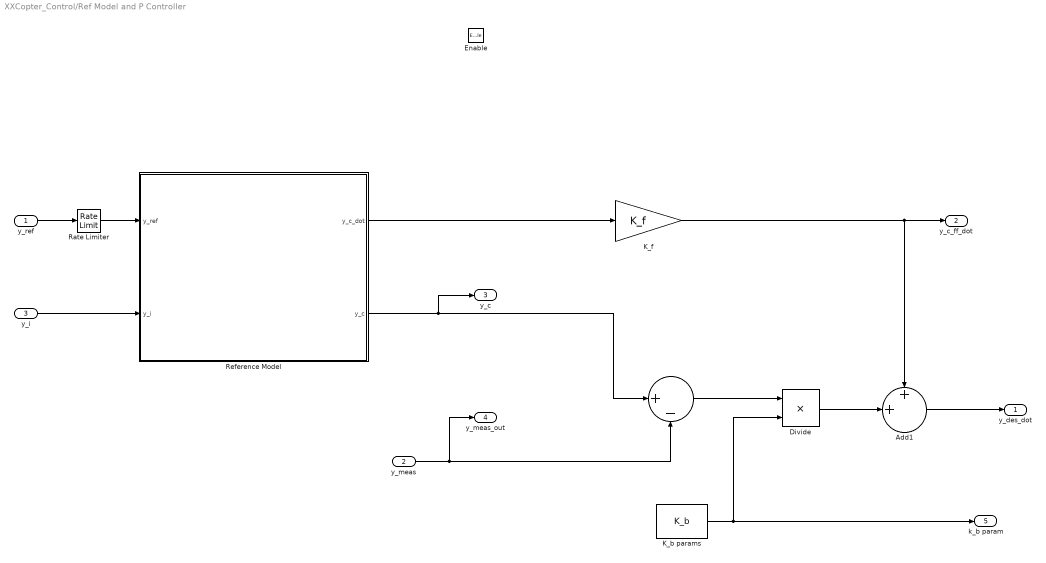
== system XXCopter_Control/Ref Model and P Controller ==
  y_ref : Inport
  y_meas : Inport  Port=2
  y_i : Inport  Port=3
  Enable : EnablePort  StatesWhenEnabling=reset
  " " : Sum  Inputs=|+-
  Add1 : Sum  Inputs=++|
  Divide : Product  Inputs=**
  K_b params : Constant  Value=K_b
  K_f : Gain  Gain=K_f
  Rate Limiter : RateLimiter  RisingSlewLimit=RisingSlewLimit  FallingSlewLimit=FallingSlewLimit  SampleTimeMode=inherited
  Reference Model : Subsystem  mask{tau=tau}
      mask prompts: tau "1st order time constant (tau)"
      mask init:
      | K_ref=1/tau;
      mask Display:
      | [y,t]=step(tf([K_ref],[1 K_ref]));
      | pos = get_param(gcb, 'Position');
      | width = pos(3) - pos(1);
      | height = pos(4) - pos(2);
      | t = t.*width/max(t);
      | y=y.*height/max(y);
      | plot(t,y);
      | 
      | 
      | text(0.5*width,0.92*height,['tau=',num2str(tau)]);
      | 
      | dpoly([K_ref],[1 K_ref], 's')
  y_des_dot : Outport
  y_c_ff_dot : Outport  Port=2
  y_c : Outport  Port=3
  y_meas_out : Outport  Port=4
  k_b param : Outport  Port=5
  wires:
  Divide/1 -> Add1/2
  K_f/1 -> Add1/1, y_c_ff_dot/1
  Reference Model/1(y_c_dot) -> K_f/1
  Add1/1 -> y_des_dot/1
  y_ref/1 -> Rate Limiter/1
  " "/1 -> Divide/1
  Reference Model/2(y_c) -> " "/1, y_c/1
  y_meas/1 -> " "/2, y_meas_out/1
  K_b params/1 -> Divide/2, k_b param/1
  y_i/1 -> Reference Model/2(y_i)
  Rate Limiter/1 -> Reference Model/1(y_ref)

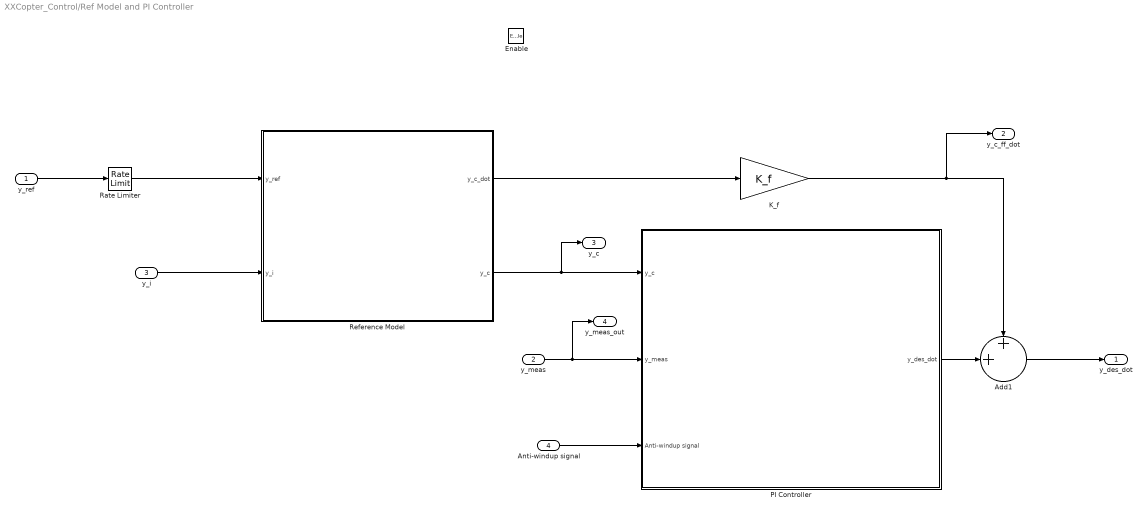
== system XXCopter_Control/Ref Model and PI Controller ==
  y_ref : Inport
  y_meas : Inport  Port=2
  y_i : Inport  Port=3
  Anti-windup signal : Inport  Port=4
  Enable : EnablePort  StatesWhenEnabling=reset
  Add1 : Sum  Inputs=++|
  K_f : Gain  Gain=K_f
  PI Controller : Subsystem  mask{K_b=K_b, f_i=f_i, f_c=f_c, K_a=K_a, delta=delta}
      mask prompts: K_b "K_b proportional term"; f_i "f_i integral term"; f_c "f_c fedfordward term"; K_a "Anti-windup gain"; delta "Integrator delay"
      mask Display:
      | if delta==0
      |     TF = tf(K_b*[f_c f_i*K_b],[1 K_b f_i*K_b^2]);
      | else
      |     s=tf('s');
      |     TF = 1/(s+delta)*K_b*(f_c*s+f_i*K_b)/(s*( 1+1/(s+delta)*K_b ) + 1/(s+delta)*f_i*K_b^2 );
      | end
      | 
      | [y,t]=step(TF);
      | S = stepinfo(y,t);
      | 
      | pos = get_param(gcb, 'Position');
      | width = pos(3) - pos(1);
      | height = pos(4) - pos(2);
      | t = t.*width/max(t);
      | y=y.*height/max(y);
      | plot(t,y);
      | 
      | S2 = stepinfo(y,t);
      | text(S2.PeakTime ,S2.Peak*0.85,['Peak time = ',num2str(S.PeakTime),'s' ]);
      | text(S2.PeakTime ,S2.Peak*0.75,['Os = ',num2str(S.Peak)]);
      | text(S2.PeakTime ,S2.Peak*0.75,['Os = ',num2str(S.Peak)]);
      | text(S2.PeakTime ,S2.Peak*0.65,['SettlingTime = ',num2str(S.SettlingTime)]);
      | 
      | text(0.1*width,0.1*height,['EXPECTED CLOSED-LOOP RESPONSE: INTEGRATION DELAY OF ',num2str(delta),'s ']);
      | 
      | [num,den] = tfdata(TF);
      | dpoly(num{:},den{:}, 's');
  Rate Limiter : RateLimiter  RisingSlewLimit=RisingSlewLimit  FallingSlewLimit=FallingSlewLimit  SampleTimeMode=inherited
  Reference Model : Subsystem  mask{tau=tau}
      mask prompts: tau "1st order time constant (tau)"
      mask init:
      | K_ref=1/tau;
      mask Display:
      | [y,t]=step(tf([K_ref],[1 K_ref]));
      | pos = get_param(gcb, 'Position');
      | width = pos(3) - pos(1);
      | height = pos(4) - pos(2);
      | t = t.*width/max(t);
      | y=y.*height/max(y);
      | plot(t,y);
      | 
      | 
      | text(0.5*width,0.92*height,['tau=',num2str(tau)]);
      | 
      | dpoly([K_ref],[1 K_ref], 's')
  y_des_dot : Outport
  y_c_ff_dot : Outport  Port=2
  y_c : Outport  Port=3
  y_meas_out : Outport  Port=4
  wires:
  y_ref/1 -> Rate Limiter/1
  Reference Model/2(y_c) -> y_c/1, PI Controller/1(y_c)
  Add1/1 -> y_des_dot/1
  Reference Model/1(y_c_dot) -> K_f/1
  K_f/1 -> y_c_ff_dot/1, Add1/1
  PI Controller/1(y_des_dot) -> Add1/2
  Anti-windup signal/1 -> PI Controller/3(Anti-windup signal)
  y_meas/1 -> y_meas_out/1, PI Controller/2(y_meas)
  y_i/1 -> Reference Model/2(y_i)
  Rate Limiter/1 -> Reference Model/1(y_ref)

== system XXCopter_Control/Rot eqs_ Get moments ==
  omega_b : Inport
  omega_dot_des : Inport  Port=2
  I_BAC : Inport  Port=3
  Cross Product : vrlib/Utilities/Cross Product
  Matrix Multiply : Product  Multiplication=Matrix(*)
  Matrix Multiply1 : Product  Multiplication=Matrix(*)
  Moment des : Sum
  Moments_des : Outport
  wires:
  Cross Product/1 -> Moment des/1
  Matrix Multiply/1 -> Cross Product/2
  omega_b/1 -> Matrix Multiply/2, Cross Product/1
  I_BAC/1 -> Matrix Multiply1/1, Matrix Multiply/1
  omega_dot_des/1 -> Matrix Multiply1/2
  Matrix Multiply1/1 -> Moment des/2
  Moment des/1 -> Moments_des/1

== system XXCopter_Control/Rotational Eq ==
  omega_b : Inport
  Moments : Inport  Port=2
  I_BAC : Inport  Port=3
  " LU Inverse" : dspinverses/ LU Inverse
  Add : Sum  Inputs=+-
  Cross Product : vrlib/Utilities/Cross Product
  Gain : Gain  Gain=-1
  Matrix Multiply : Product  Multiplication=Matrix(*)
  Matrix Multiply1 : Product  Multiplication=Matrix(*)
  omega_dot : Outport
  wires:
  I_BAC/1 -> " LU Inverse"/1, Matrix Multiply/1
  omega_b/1 -> Cross Product/1, Matrix Multiply/2
  Matrix Multiply/1 -> Cross Product/2
  Cross Product/1 -> Gain/1
  Moments/1 -> Add/1
  Gain/1 -> Add/2
  Add/1 -> Matrix Multiply1/2
  " LU Inverse"/1 -> Matrix Multiply1/1
  Matrix Multiply1/1 -> omega_dot/1

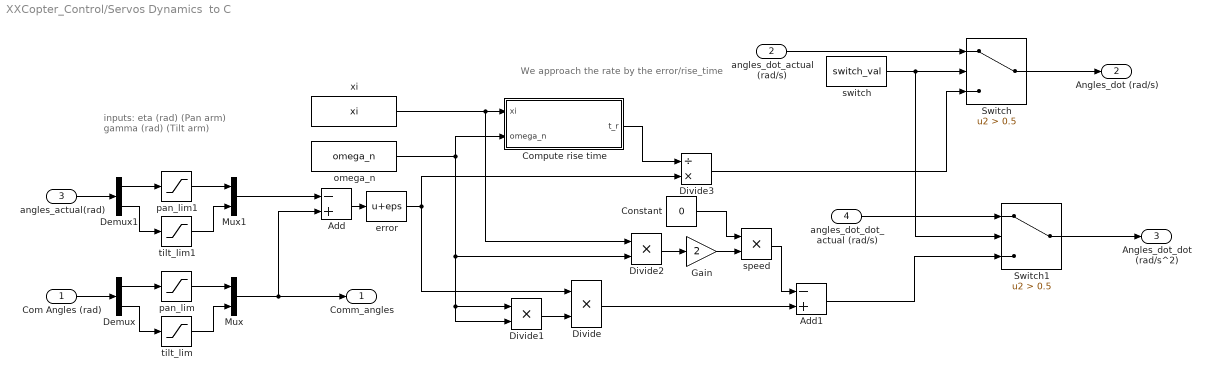
== system XXCopter_Control/Servos Dynamics  to C ==
  note: We approach the rate by the error/rise_time
  note: inputs:
      | eta (rad)  (Pan arm)
      | gamma (rad)  (Tilt arm)
  Com Angles (rad) : Inport
  angles_dot_actual (rad/s) : Inport  Port=2
  angles_actual(rad) : Inport  Port=3
  angles_dot_dot_actual (rad/s) : Inport  Port=4
  Add : Sum  Inputs=-+
  Add1 : Sum  Inputs=-+
  Compute rise time : MATLAB Function  TreatAsAtomicUnit=on
  Constant : Constant  Value=0
  Demux : Demux  Outputs=2
  Demux1 : Demux  Outputs=2
  Divide : Product  Inputs=**
  Divide1 : Product  Inputs=**
  Divide2 : Product  Inputs=**
  Divide3 : Product  Inputs=/*
  Gain : Gain  Gain=2
  Mux : Mux  Inputs=2
  Mux1 : Mux  Inputs=2
  Switch : Switch  Criteria=u2 > Threshold  Threshold=0.5
  Switch1 : Switch  Criteria=u2 > Threshold  Threshold=0.5
  error : Bias  Bias=eps
  omega_n : Constant  Value=omega_n
  pan_lim : Saturate  UpperLimit=eta_sup_lim  LowerLimit=eta_inf_lim
  pan_lim1 : Saturate  UpperLimit=eta_sup_lim  LowerLimit=eta_inf_lim
  speed : Product  Inputs=**
  switch : Constant  Value=switch_val
  tilt_lim : Saturate  UpperLimit=gamma_sup_lim  LowerLimit=gamma_inf_lim
  tilt_lim1 : Saturate  UpperLimit=gamma_sup_lim  LowerLimit=gamma_inf_lim
  xi : Constant  Value=xi
  Comm_angles : Outport
  Angles_dot (rad/s) : Outport  Port=2
  Angles_dot_dot (rad/s^2) : Outport  Port=3
  wires:
  Mux1/1 -> Add/1
  Mux/1 -> Comm_angles/1, Add/2
  Add/1 -> error/1
  Divide1/1 -> Divide/2
  xi/1 -> Divide2/1, Compute rise time/1(xi)
  Divide2/1 -> Gain/1
  Divide/1 -> Add1/2
  Gain/1 -> speed/2
  speed/1 -> Add1/1
  Com Angles (rad)/1 -> Demux/1
  Demux/1 -> pan_lim/1
  pan_lim/1 -> Mux/1
  Demux/2 -> tilt_lim/1
  tilt_lim/1 -> Mux/2
  angles_actual(rad)/1 -> Demux1/1
  Demux1/1 -> pan_lim1/1
  pan_lim1/1 -> Mux1/1
  Demux1/2 -> tilt_lim1/1
  tilt_lim1/1 -> Mux1/2
  error/1 -> Divide/1, Divide3/2
  omega_n/1 -> Divide1/2, Divide1/1, Divide2/2, Compute rise time/2(omega_n)
  Compute rise time/1(t_r) -> Divide3/1
  Divide3/1 -> Switch/3
  Constant/1 -> speed/1
  switch/1 -> Switch/2, Switch1/2
  Switch/1 -> Angles_dot (rad/s)/1
  angles_dot_actual (rad/s)/1 -> Switch/1
  Switch1/1 -> Angles_dot_dot (rad/s^2)/1
  angles_dot_dot_actual (rad/s)/1 -> Switch1/1
  Add1/1 -> Switch1/3

== system XXCopter_Control/Signal2PWM ==
  Signal : Inport
  Add : Sum  Inputs=+-
  Add1 : Sum  Inputs=+-
  Add2 : Sum  Inputs=+-
  Add3 : Sum
  Divide : Product  Inputs=*/
  Divide1 : Product  Inputs=**
  down_PWM : Constant  Value=c
  down_signal : Constant  Value=d
  up_PWM : Constant  Value=a
  up_signal : Constant  Value=b
  PWM_us : Outport
  wires:
  Signal/1 -> Add/1
  down_signal/1 -> Add/2, Add1/2
  up_signal/1 -> Add1/1
  Add1/1 -> Divide/2
  Add/1 -> Divide/1
  up_PWM/1 -> Add2/1
  down_PWM/1 -> Add3/1, Add2/2
  Divide/1 -> Divide1/2
  Add2/1 -> Divide1/1
  Divide1/1 -> Add3/2
  Add3/1 -> PWM_us/1

== system XXCopter_Control/Transl Eqs_ Get forces ==
  A_des : Inport
  Vb : Inport  Port=2
  omega_b : Inport  Port=3
  omega_b_dot : Inport  Port=4
  m : Inport  Port=5
  CG : Inport  Port=6
  Add : Sum  Inputs=++++
  Cross Product{,1..3} (4 alike) : vrlib/Utilities/Cross Product
  Product : Product  RndMeth=Zero
  Forces_des : Outport
  wires:
  Add/1 -> Product/1
  Cross Product/1 -> Add/3
  Cross Product3/1 -> Add/2
  Cross Product2/1 -> Add/1
  omega_b_dot/1 -> Cross Product3/1
  Cross Product1/1 -> Cross Product2/2
  CG/1 -> Cross Product1/2, Cross Product3/2
  Vb/1 -> Cross Product/2
  omega_b/1 -> Cross Product/1, Cross Product1/1, Cross Product2/1
  m/1 -> Product/2
  A_des/1 -> Add/4
  Product/1 -> Forces_des/1

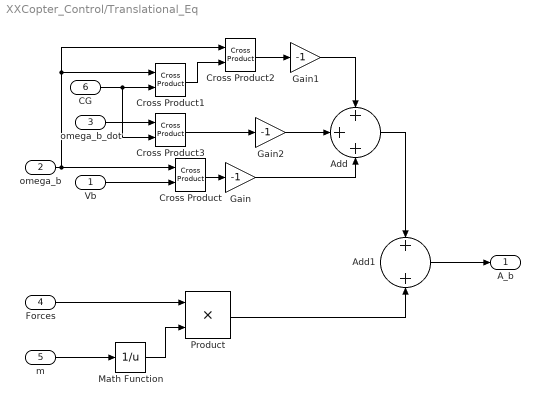
== system XXCopter_Control/Translational_Eq ==
  Vb : Inport
  omega_b : Inport  Port=2
  omega_b_dot : Inport  Port=3
  Forces : Inport  Port=4
  m : Inport  Port=5
  CG : Inport  Port=6
  Add : Sum  Inputs=+++
  Add1 : Sum
  Cross Product{,1..3} (4 alike) : vrlib/Utilities/Cross Product
  Gain : Gain  Gain=-1
  Gain1 : Gain  Gain=-1
  Gain2 : Gain  Gain=-1
  Math Function : Math  Operator=reciprocal  SaturateOnIntegerOverflow=on
  Product : Product  RndMeth=Zero
  A_b : Outport
  wires:
  m/1 -> Math Function/1
  Math Function/1 -> Product/2
  Forces/1 -> Product/1
  omega_b/1 -> Cross Product2/1, Cross Product1/1, Cross Product/1
  Vb/1 -> Cross Product/2
  Cross Product/1 -> Gain/1
  CG/1 -> Cross Product3/2, Cross Product1/2
  Cross Product1/1 -> Cross Product2/2
  Cross Product2/1 -> Gain1/1
  omega_b_dot/1 -> Cross Product3/1
  Cross Product3/1 -> Gain2/1
  Gain1/1 -> Add/1
  Gain2/1 -> Add/2
  Gain/1 -> Add/3
  Product/1 -> Add1/2
  Add/1 -> Add1/1
  Add1/1 -> A_b/1

== system XXCopter_Control/2D vec norm/norm^2rm ==
  v : Inport
  Demux : Demux  Outputs=2
  Product : Product
  Product1 : Product
  Sum : Sum  Inputs=2
  norm(v) : Outport
  wires:
  v/1 -> Demux/1
  Sum/1 -> norm(v)/1
  Product/1 -> Sum/1
  Product1/1 -> Sum/2
  Demux/1 -> Product/1, Product/2
  Demux/2 -> Product1/2, Product1/1

== system XXCopter_Control/3D vec norm/norm^2rm ==
  v : Inport
  Demux : Demux  Outputs=3
  Product : Product
  Product1 : Product
  Product2 : Product
  Sum : Sum  Inputs=3
  norm(v) : Outport
  wires:
  Demux/2 -> Product1/2, Product1/1
  Demux/1 -> Product/2, Product/1
  Product1/1 -> Sum/2
  Product/1 -> Sum/1
  Sum/1 -> norm(v)/1
  v/1 -> Demux/1
  Demux/3 -> Product2/2, Product2/1
  Product2/1 -> Sum/3

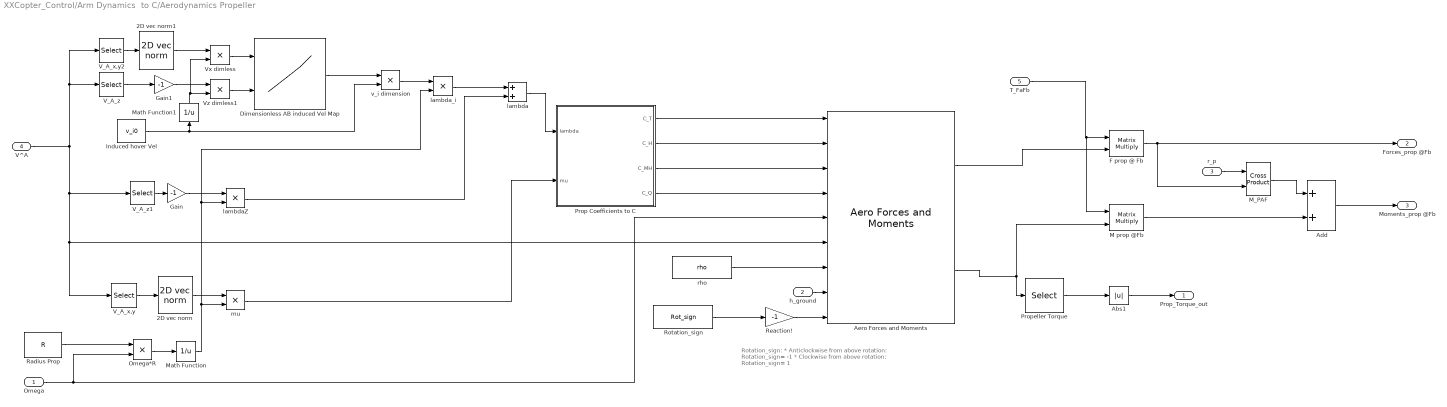
== system XXCopter_Control/Arm Dynamics  to C/Aerodynamics Propeller ==
  note: Rotation_sign:
      |
      | * Anticlockwise from above rotation: Rotation_sign= -1
      | * Clockwise from above rotation: Rotation_sign= 1
  Omega : Inport
  h_ground : Inport  Port=2
  r_p : Inport  Port=3
  V^A : Inport  Port=4
  T_FaFb : Inport  Port=5
  2D vec norm : XXCopter_Control/2D vec norm
  2D vec norm1 : XXCopter_Control/2D vec norm
  Abs1 : Abs
  Add : Sum
  "Aero Forces and Moments " : XXCopter_Control/Aero Forces and Moments 
  Dimensionless AB induced Vel Map : Lookup_n-D  BreakpointsForDimension1=Vx_adim  BreakpointsForDimension2=Vz_adim  BreakpointsForDimension3=[5, 7]  Table=v_i_adim  TableDataTypeStr=single  IntermediateResultsDataTypeStr=single  ExtrapMethod=Clip  RemoveProtectionInput=on  OutDataTypeStr=single  RndMeth=Zero  FractionDataTypeStr=single  InputSameDT=on
  F prop @ Fb : Product  Multiplication=Matrix(*)
  Gain : Gain  Gain=-1
  Gain1 : Gain  Gain=-1
  Induced hover Vel : Constant  Value=v_i0
  M prop @Fb : Product  Multiplication=Matrix(*)
  M_PAF : vrlib/Utilities/Cross Product
  Math Function : Math  Operator=reciprocal  SaturateOnIntegerOverflow=on
  Math Function1 : Math  Operator=reciprocal  SaturateOnIntegerOverflow=on
  Omega*R : Product  Inputs=**
  Prop Coefficients to C : MATLAB Function  TreatAsAtomicUnit=on
  Propeller Torque : Selector  IndexMode=Zero-based  InputPortWidth=3  Indices=2
  Radius Prop : Constant  Value=R  OutDataTypeStr=double
  Reaction! : Gain  Gain=-1
  Rotation_sign : Constant  Value=Rot_sign
  V_A_x,y : Selector  IndexMode=Zero-based  InputPortWidth=3  Indices=[0,1]
  V_A_x,y2 : Selector  IndexMode=Zero-based  InputPortWidth=3  Indices=[0,1]
  V_A_z : Selector  IndexMode=Zero-based  InputPortWidth=3  Indices=2
  V_A_z1 : Selector  IndexMode=Zero-based  InputPortWidth=3  Indices=2
  Vx dimless : Product  Inputs=**  OutDataTypeStr=double
  Vz dimless1 : Product  Inputs=**  OutDataTypeStr=double
  lambda : Sum
  lambdaZ : Product  Inputs=**
  lambda_i : Product  Inputs=**
  mu : Product  Inputs=**
  rho : Constant  Value=rho
  v_i dimension : Product  Inputs=**
  Prop_Torque_out : Outport
  Forces_prop @Fb : Outport  Port=2
  Moments_prop @Fb : Outport  Port=3
  wires:
  Radius Prop/1 -> Omega*R/1
  V_A_x,y/1 -> 2D vec norm/1
  2D vec norm/1 -> mu/1
  Omega*R/1 -> Math Function/1
  Vx dimless/1 -> Dimensionless AB induced Vel Map/1
  V_A_x,y2/1 -> 2D vec norm1/1
  Vz dimless1/1 -> Dimensionless AB induced Vel Map/2
  V_A_z/1 -> Gain1/1
  Induced hover Vel/1 -> v_i dimension/2, Math Function1/1
  Dimensionless AB induced Vel Map/1 -> v_i dimension/1
  v_i dimension/1 -> lambda_i/1
  V_A_z1/1 -> Gain/1
  Gain/1 -> lambdaZ/1
  lambda_i/1 -> lambda/1
  lambdaZ/1 -> lambda/2
  Gain1/1 -> Vz dimless1/1
  lambda/1 -> Prop Coefficients to C/1(lambda)
  Prop Coefficients to C/1(C_T) -> "Aero Forces and Moments "/1
  Prop Coefficients to C/2(C_H) -> "Aero Forces and Moments "/2
  Prop Coefficients to C/3(C_MH) -> "Aero Forces and Moments "/3
  V^A/1 -> V_A_z1/1, "Aero Forces and Moments "/6, V_A_x,y/1, V_A_x,y2/1, V_A_z/1
  Omega/1 -> "Aero Forces and Moments "/5, Omega*R/2
  "Aero Forces and Moments "/2 -> M prop @Fb/2, Propeller Torque/1
  Add/1 -> Moments_prop @Fb/1
  h_ground/1 -> "Aero Forces and Moments "/8
  Rotation_sign/1 -> Reaction!/1
  Propeller Torque/1 -> Abs1/1
  T_FaFb/1 -> M prop @Fb/1, F prop @ Fb/1
  "Aero Forces and Moments "/1 -> F prop @ Fb/2
  F prop @ Fb/1 -> M_PAF/2, Forces_prop @Fb/1
  r_p/1 -> M_PAF/1
  M_PAF/1 -> Add/1
  M prop @Fb/1 -> Add/2
  Abs1/1 -> Prop_Torque_out/1
  2D vec norm1/1 -> Vx dimless/1
  mu/1 -> Prop Coefficients to C/2(mu)
  Prop Coefficients to C/4(C_Q) -> "Aero Forces and Moments "/4
  Reaction!/1 -> "Aero Forces and Moments "/9
  Math Function/1 -> mu/2, lambdaZ/2, lambda_i/2
  Math Function1/1 -> Vz dimless1/2, Vx dimless/2
  rho/1 -> "Aero Forces and Moments "/7

== system XXCopter_Control/GCS params safemode/Sample&Hold ==
  In1 : Inport
  Trigger : TriggerPort
  Out1 : Outport
  wires:
  In1/1 -> Out1/1

== system XXCopter_Control/Normalize 4D vector/4D vec norm ==
  v : Inport
  norm^2rm : Subsystem  TreatAsAtomicUnit=on
  sqrt : Sqrt  AlgorithmType=Newton-Raphson  SaturateOnIntegerOverflow=on
  norm(v) : Outport
  wires:
  sqrt/1 -> norm(v)/1
  norm^2rm/1(norm(v)) -> sqrt/1
  v/1 -> norm^2rm/1(v)

== system XXCopter_Control/Ref Model and P Controller/Reference Model ==
  y_ref : Inport
  y_i : Inport  Port=2
  Add : Sum  Inputs=|+-
  Integrator : Integrator  InitialConditionSource=external
  K_ref : Gain  Gain=K_ref
  y_c_dot : Outport
  y_c : Outport  Port=2
  wires:
  y_i/1 -> Integrator/2
  Integrator/1 -> Add/2, y_c/1
  K_ref/1 -> Integrator/1, y_c_dot/1
  Add/1 -> K_ref/1
  y_ref/1 -> Add/1

== system XXCopter_Control/Ref Model and PI Controller/PI Controller ==
  y_c : Inport
  y_meas : Inport  Port=2
  Anti-windup signal : Inport  Port=3
  " " : Sum  Inputs=++-
  " 1" : Sum  Inputs=|++
  Add : Sum  Inputs=|+-
  Integrator : Integrator
  K_a : Gain  Gain=K_a
  K_b : Gain  Gain=K_b
  f_c : Gain  Gain=f_c
  f_i*K_b : Gain  Gain=f_i*K_b
  y_des_dot : Outport
  wires:
  f_i*K_b/1 -> " 1"/1
  Add/1 -> f_i*K_b/1
  K_b/1 -> y_des_dot/1
  y_meas/1 -> " "/3, Add/2
  y_c/1 -> f_c/1, Add/1
  Integrator/1 -> " "/2
  f_c/1 -> " "/1
  " "/1 -> K_b/1
  Anti-windup signal/1 -> K_a/1
  " 1"/1 -> Integrator/1
  K_a/1 -> " 1"/2

== system XXCopter_Control/Ref Model and PI Controller/Reference Model ==
  y_ref : Inport
  y_i : Inport  Port=2
  Add : Sum  Inputs=|+-
  Integrator : Integrator  InitialConditionSource=external
  K_ref : Gain  Gain=K_ref
  y_c_dot : Outport
  y_c : Outport  Port=2
  wires:
  y_ref/1 -> Add/1
  Add/1 -> K_ref/1
  K_ref/1 -> Integrator/1, y_c_dot/1
  Integrator/1 -> y_c/1, Add/2
  y_i/1 -> Integrator/2
